simulink model "ParachuteSim"  (R2024b)
settings: Solver=VariableStepAuto  StartTime=0.0  StopTime=500  FixedStep=1/300  MaxStep=0.1  RelTol=1e-3  EnableMultiTasking=on
PreLoadFcn:
  | % initialize values allowing model to run without Live Script
  | windDisturbance = true;
  | windSeed = randi(100,1);
  | headingInitial = 45;
  | latInitial = 43.5319;
  | longInitial = 1.2438;
  | XeInitial = 0;
  | YeInitial = 0;
  | ZeInitial = 2000;
  | UInitialMPS = 65.277777777777790;
  | VInitialMPS = 0;
  | WInitialMPS = 0;
  | hOpening = 500;
  | packageMass = 130;
  | area = 115;
  | mass = 165;
  | velocity = 6;
  | g = 9.81;
  | rho = 1.229;
  | Cd = 2*mass*g/(rho*(velocity^2)*area);
undefined symbols (not defined in the file): Earth, F, Light, MIL, WGS84
libraries: aerolibwind2 x3, simulink x2, aerolibatmos2 x1, aerolibtransform2 x1, shared6dof x1
CloseFcn:
  | clear windDisturbance windSeed;
  | clear headingInitial latInitial longInitial;
  | clear XeInitial YeInitial ZeInitial;
  | clear UInitialMPS VInitialMPS WInitialMPS;
  | clear hOpening packageMass;
  | clear area mass velocity g rho Cd;
settings Model: Creator=The MathWorks, Inc.  LastModifiedBy=franklinho
settings SolverCC: AutoInsertRateTranBlk=on
settings OptimizationCC: ReuseModelBlockBuffer=off
settings DebuggingCC: UnconnectedInputMsg=warning  UnconnectedOutputMsg=warning  UnconnectedLineMsg=warning
settings ModelReferenceCC: EnableRefExpFcnMdlSchedulingChecks=on
settings RTWCC: GPUComputeCapability=3.5  DLArmComputeVersion=19.05

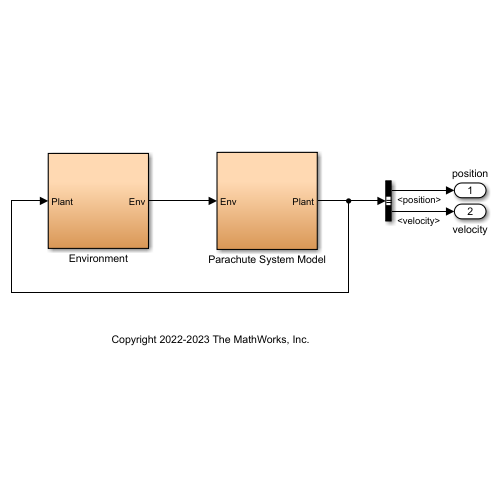
[thumbnail: Simulink's stored preview of the top-level diagram]
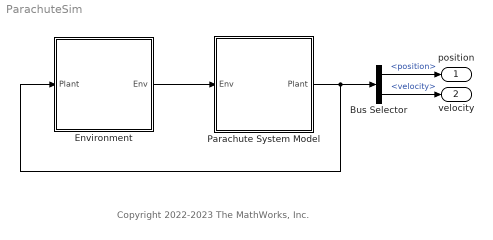
== system ParachuteSim ==
  note: Copyright 2022-2023 The MathWorks, Inc.
  Bus Selector : BusSelector  OutputSignals=position,velocity
  Environment : Subsystem
  Parachute System Model : Subsystem
  position : Outport
  velocity : Outport  Port=2
  wires:
  Parachute System Model/1(Plant) -> Environment/1(Plant), Bus Selector/1
  Environment/1(Env) -> Parachute System Model/1(Env)
  Bus Selector/1 -> position/1  "<position>"
  Bus Selector/2 -> velocity/1  "<velocity>"

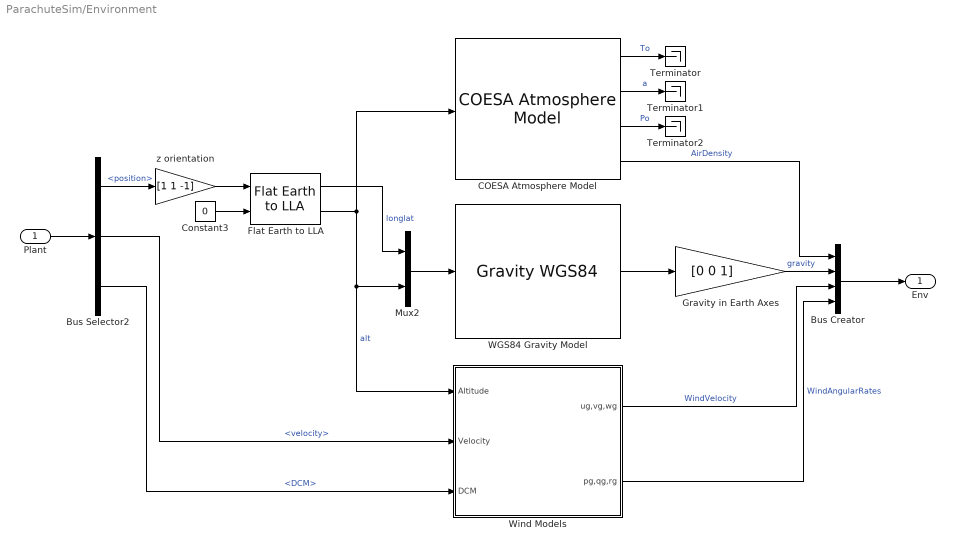
== system ParachuteSim/Environment ==
  Plant : Inport
  Bus Creator : BusCreator  Inputs=4
  Bus Selector2 : BusSelector  OutputSignals=position,velocity,DCM
  COESA Atmosphere Model : aerolibatmos2/COESA Atmosphere Model  units=Metric (MKS)  spec=1976 COESA-extended U.S. Standard Atmosphere  model=Profile  profile_var=High temperature  profile_percent=1%  profile_alt=5 km (16404 ft)  envelope_var=High temperature  envelope_percent=1%  action=None
  Constant3 : Constant  Value=0
  Flat Earth to LLA : aerolibtransform2/Flat Earth to LLA  units=Metric (MKS)  ptype=Earth (WGS84)  F=1/298.257223563  R=6378137  refPosPort=off  LL0=[latInitial, longInitial]  psi=headingInitial
  Gravity in Earth Axes : Gain  Gain=[0 0 1]  SaturateOnIntegerOverflow=on  OutDataTypeStr=Inherit: Same as input  ParamDataTypeStr=Inherit: Same as input
  Mux2 : Mux  Inputs=2
  Terminator : Terminator
  Terminator1 : Terminator
  Terminator2 : Terminator
  "WGS84 Gravity Model  " : GravityWGS84  action=None
  Wind Models : Subsystem
  z orientation : Gain  Gain=[1 1 -1]
  Env : Outport
  wires:
  Bus Selector2/2 -> Wind Models/2(Velocity)  "<velocity>"
  Bus Selector2/1 -> z orientation/1  "<position>"
  Bus Creator/1 -> Env/1
  Plant/1 -> Bus Selector2/1
  "WGS84 Gravity Model  "/1 -> Gravity in Earth Axes/1
  Mux2/1 -> "WGS84 Gravity Model  "/1
  Constant3/1 -> Flat Earth to LLA/2
  Flat Earth to LLA/1 -> Mux2/1  "longlat"
  Gravity in Earth Axes/1 -> Bus Creator/2  "gravity"
  z orientation/1 -> Flat Earth to LLA/1
  COESA Atmosphere Model/1 -> Terminator/1  "To"
  COESA Atmosphere Model/2 -> Terminator1/1  "a"
  COESA Atmosphere Model/3 -> Terminator2/1  "Po"
  COESA Atmosphere Model/4 -> Bus Creator/1  "AirDensity"
  Flat Earth to LLA/2 -> COESA Atmosphere Model/1, Wind Models/1(Altitude), Mux2/2  "alt"
  Bus Selector2/3 -> Wind Models/3(DCM)  "<DCM>"
  Wind Models/1(ug,vg,wg) -> Bus Creator/3  "WindVelocity"
  Wind Models/2(pg,qg,rg) -> Bus Creator/4  "WindAngularRates"

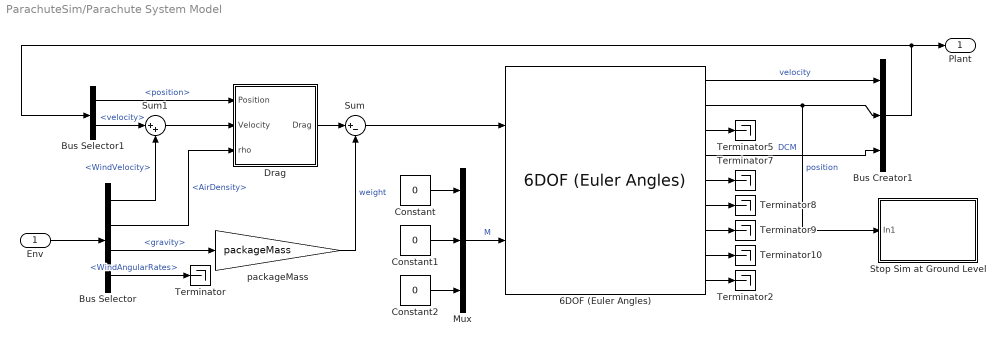
== system ParachuteSim/Parachute System Model ==
  Env : Inport
  6DOF (Euler Angles) : shared6dof/6DOF (Euler Angles)  units=Metric (MKS)  mtype=Fixed  rep=Euler Angles  xme_0=[XeInitial,YeInitial,ZeInitial]  Vm_0=[UInitialMPS,VInitialMPS,WInitialMPS]  eul_0=[0 0 0]  pm_0=[0 0 0]  mass_0=packageMass  mass_e=0.5  mass_f=2.0  inertia=eye(3)  inertia_e=eye(3)  inertia_f=2*eye(3)  k_quat=1.0  vre_flag=on  abi_flag=on  aMode=0  xme_statename=''  Vm_statename=''  eul_statename=''  quat_statename=''  pm_statename=''  mass_statename=''
  Bus Creator1 : BusCreator  Inputs=3
  Bus Selector : BusSelector  OutputSignals=WindVelocity,AirDensity,gravity,WindAngularRates
  Bus Selector1 : BusSelector  OutputSignals=position,velocity
  Constant : Constant  Value=0
  Constant1 : Constant  Value=0
  Constant2 : Constant  Value=0
  Drag : Subsystem
  Mux : Mux  Inputs=3
  Stop Sim at Ground Level : Subsystem
  Sum : Sum  Inputs=|+-
  Sum1 : Sum  Inputs=|++
  Terminator{,2,5,7..10} (7 alike) : Terminator
  packageMass : Gain  Gain=packageMass
  Plant : Outport
  wires:
  Sum/1 -> 6DOF (Euler Angles)/1
  6DOF (Euler Angles)/8 -> Terminator10/1
  6DOF (Euler Angles)/5 -> Terminator7/1
  6DOF (Euler Angles)/3 -> Terminator5/1
  6DOF (Euler Angles)/4 -> Bus Creator1/3  "DCM"
  6DOF (Euler Angles)/7 -> Terminator9/1
  6DOF (Euler Angles)/6 -> Terminator8/1
  6DOF (Euler Angles)/1 -> Bus Creator1/1  "velocity"
  6DOF (Euler Angles)/2 -> Stop Sim at Ground Level/1(In1), Bus Creator1/2  "position"
  6DOF (Euler Angles)/9 -> Terminator2/1
  Bus Creator1/1 -> Plant/1, Bus Selector1/1
  Drag/1(Drag) -> Sum/1
  Constant1/1 -> Mux/2
  Mux/1 -> 6DOF (Euler Angles)/2  "M"
  Constant2/1 -> Mux/3
  Constant/1 -> Mux/1
  Env/1 -> Bus Selector/1
  Bus Selector/2 -> Drag/3(rho)  "<AirDensity>"
  Bus Selector/3 -> packageMass/1  "<gravity>"
  Bus Selector1/1 -> Drag/1(Position)  "<position>"
  Bus Selector/4 -> Terminator/1  "<WindAngularRates>"
  Sum1/1 -> Drag/2(Velocity)
  Bus Selector1/2 -> Sum1/1  "<velocity>"
  Bus Selector/1 -> Sum1/2  "<WindVelocity>"
  packageMass/1 -> Sum/2  "weight"

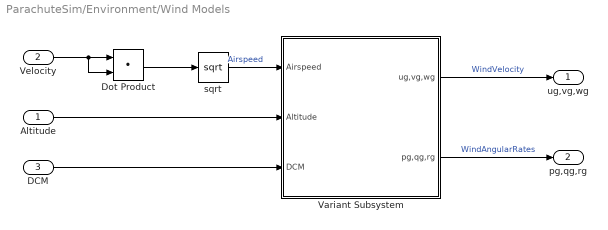
== system ParachuteSim/Environment/Wind Models ==
  Altitude : Inport
  Velocity : Inport  Port=2
  DCM : Inport  Port=3
  Dot Product : DotProduct  InputSameDT=off  OutDataTypeStr=Inherit: Inherit via internal rule
  Variant Subsystem : Subsystem  Variant=on
  sqrt : Sqrt
  ug,vg,wg : Outport  Unit=m/s  VectorParamsAs1DForOutWhenUnconnected=off
  pg,qg,rg : Outport  Port=2  Unit=rad/second  VectorParamsAs1DForOutWhenUnconnected=off
  wires:
  DCM/1 -> Variant Subsystem/3(DCM)
  Altitude/1 -> Variant Subsystem/2(Altitude)
  sqrt/1 -> Variant Subsystem/1(Airspeed)  "Airspeed"
  Dot Product/1 -> sqrt/1
  Variant Subsystem/2(pg,qg,rg) -> pg,qg,rg/1  "WindAngularRates"
  Variant Subsystem/1(ug,vg,wg) -> ug,vg,wg/1  "WindVelocity"
  Velocity/1 -> Dot Product/2, Dot Product/1

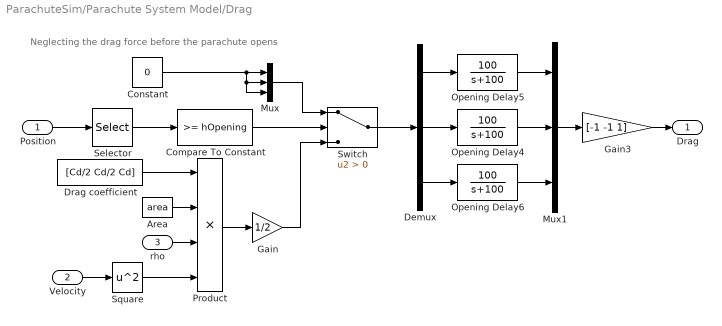
== system ParachuteSim/Parachute System Model/Drag ==
  note: Neglecting the drag force before the parachute opens
  Position : Inport
  Velocity : Inport  Port=2
  rho : Inport  Port=3
  Area : Constant  Value=area
  Compare To Constant : simulink/Logic and Bit Operations/Compare To Constant  relop=>=  const=hOpening  OutDataTypeStr=boolean
  Constant : Constant  Value=0
  Demux : Demux  Outputs=3
  Drag coefficient : Constant  Value=[Cd/2 Cd/2 Cd]
  Gain : Gain  Gain=1/2
  Gain3 : Gain  Gain=[-1 -1 1]
  Mux : Mux  Inputs=3
  Mux1 : Mux  Inputs=3
  Opening Delay4 : TransferFcn  Numerator=[100]  Denominator=[1 100]
  Opening Delay5 : TransferFcn  Numerator=[100]  Denominator=[1 100]
  Opening Delay6 : TransferFcn  Numerator=[100]  Denominator=[1 100]
  Product : Product  Inputs=4
  Selector : Selector  InputPortWidth=3  IndexOptions=Index vector (dialog)  Indices=[3]  OutputSizes=1
  Square : Math  Operator=square
  Switch : Switch  Criteria=u2 > Threshold  SaturateOnIntegerOverflow=off  InputSameDT=off
  Drag : Outport
  wires:
  Velocity/1 -> Square/1
  Product/1 -> Gain/1
  Compare To Constant/1 -> Switch/2
  Position/1 -> Selector/1
  Gain/1 -> Switch/3
  Mux/1 -> Switch/1
  Constant/1 -> Mux/3, Mux/2, Mux/1
  Switch/1 -> Demux/1
  Demux/3 -> Opening Delay6/1
  Selector/1 -> Compare To Constant/1
  Mux1/1 -> Gain3/1
  Demux/1 -> Opening Delay5/1
  Demux/2 -> Opening Delay4/1
  Gain3/1 -> Drag/1
  Opening Delay5/1 -> Mux1/1
  Opening Delay6/1 -> Mux1/3
  Opening Delay4/1 -> Mux1/2
  rho/1 -> Product/3
  Square/1 -> Product/4
  Area/1 -> Product/2
  Drag coefficient/1 -> Product/1

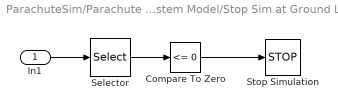
== system ParachuteSim/Parachute System Model/Stop Sim at Ground Level ==
  In1 : Inport
  Compare To Zero : simulink/Logic and Bit Operations/Compare To Zero  relop=<=  OutDataTypeStr=boolean
  Selector : Selector  InputPortWidth=3  IndexOptions=Index vector (dialog)  Indices=[3]  OutputSizes=1
  Stop Simulation : Stop
  wires:
  Compare To Zero/1 -> Stop Simulation/1
  In1/1 -> Selector/1
  Selector/1 -> Compare To Zero/1

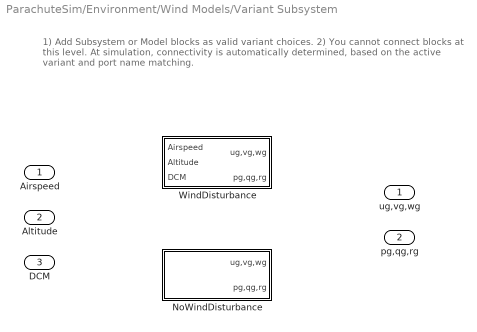
== system ParachuteSim/Environment/Wind Models/Variant Subsystem ==
  note: 1) Add Subsystem or Model blocks as valid variant choices.
      | 2) You cannot connect blocks at this level. At simulation, connectivity is automatically
      | determined, based on the active variant and port name matching.
  Airspeed : Inport
  Altitude : Inport  Port=2
  DCM : Inport  Port=3
  NoWindDisturbance : Subsystem  VariantControl=windDisturbance==false
  WindDisturbance : Subsystem  VariantControl=windDisturbance==true
  ug,vg,wg : Outport
  pg,qg,rg : Outport  Port=2

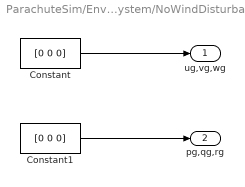
== system ParachuteSim/Environment/Wind Models/Variant Subsystem/NoWindDisturbance ==
  Constant : Constant  Value=[0 0 0]
  Constant1 : Constant  Value=[0 0 0]
  ug,vg,wg : Outport
  pg,qg,rg : Outport  Port=2  Unit=rad/second  VectorParamsAs1DForOutWhenUnconnected=off
  wires:
  Constant/1 -> ug,vg,wg/1
  Constant1/1 -> pg,qg,rg/1

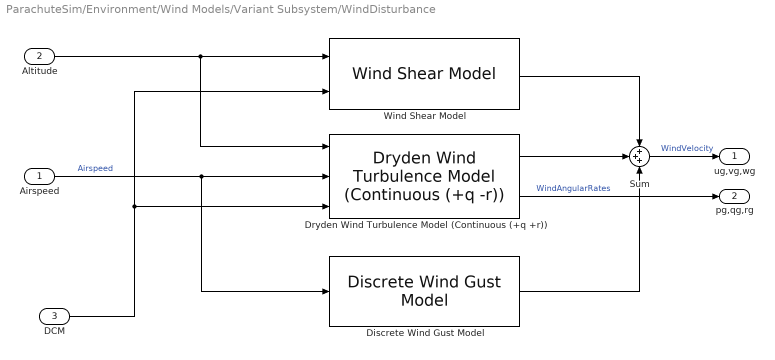
== system ParachuteSim/Environment/Wind Models/Variant Subsystem/WindDisturbance ==
  Airspeed : Inport
  Altitude : Inport  Port=2
  DCM : Inport  Port=3
  Discrete Wind Gust Model : aerolibwind2/Discrete Wind Gust Model  units=Metric (MKS)  Gx=on  Gy=on  Gz=off  t_0=windSeed  d_m=[120 120 80]  v_m=[0 0 0]
  Dryden Wind Turbulence Model (Continuous (+q +r)) : aerolibwind2/Dryden Wind Turbulence Model  (Continuous (+q -r))  units=Metric (MKS)  spec=MIL-F-8785C  model=Continuous Dryden (+q -r)  W20=1  Wdeg=0  TurbProb=10^-2 - Light  L_high=533.4  Wingspan=4  ts=0.1  Seed=[23341 23342 23343 23344]  T_on=on
  Sum : Sum  Inputs=+++  InputSameDT=on  SaturateOnIntegerOverflow=on  OutDataTypeStr=Inherit: Same as first input
  Wind Shear Model : aerolibwind2/Wind Shear Model  units=Metric (MKS)  phase=Category C - Terminal Flight Phase  W_20=1  Wdeg=0
  ug,vg,wg : Outport
  pg,qg,rg : Outport  Port=2  Unit=rad/second  VectorParamsAs1DForOutWhenUnconnected=off
  wires:
  Altitude/1 -> Dryden Wind Turbulence Model (Continuous (+q +r))/1, Wind Shear Model/1
  Airspeed/1 -> Discrete Wind Gust Model/1, Dryden Wind Turbulence Model (Continuous (+q +r))/2  "Airspeed"
  Wind Shear Model/1 -> Sum/1
  Dryden Wind Turbulence Model (Continuous (+q +r))/1 -> Sum/2
  DCM/1 -> Dryden Wind Turbulence Model (Continuous (+q +r))/3, Wind Shear Model/2
  Discrete Wind Gust Model/1 -> Sum/3
  Sum/1 -> ug,vg,wg/1  "WindVelocity"
  Dryden Wind Turbulence Model (Continuous (+q +r))/2 -> pg,qg,rg/1  "WindAngularRates"
